simulink model "Simulacion_FIiltro_Adaptado1"  (R2020b)
settings: Solver=ode45  StartTime=0.0  StopTime=3*Tb  RelTol=1e-3  EnableMultiTasking=on
values from neighbouring files (symbols this model uses):
  Canal = 1/600    (= 0.00166666666667)    [filtroadaptado.m]
  Tb = Ts    (= 0.0276)    [filtroadaptado.m]
libraries: simulink_extras x1, commnoisgen2 x1
settings Model: Creator=Dario  LastModifiedBy=Agustin
settings DataIOCC: LimitDataPoints=on  SaveFormat=Array  ReturnWorkspaceOutputs=off
settings OptimizationCC: LifeSpan=inf
settings DebuggingCC: UnderspecifiedInitializationDetection=Classic  MergeDetectMultiDrivingBlocksExec=none  SolverPrmCheckMsg=warning  StateNameClashWarn=warning  SFUnexpectedBacktrackingDiag=warning  SFNoUnconditionalDefaultTransitionDiag=warning  SFExecutionAtInitializationDiag=none  ArithmeticOperatorsInVariantConditions=warning
settings HardwareCC: ProdBitPerPointer=32  ProdBitPerSizeT=32  ProdBitPerPtrDiffT=32  ProdLargestAtomicFloat=None  ProdIntDivRoundTo=Undefined  ProdEndianess=Unspecified  ProdWordSize=32  ProdHWDeviceType=32-bit Generic
settings ModelReferenceCC: PropagateSignalLabelsOutOfModel=off
settings SFSimCC: SimUseLocalCustomCode=off  CustomCodeUndefinedFunction=UseInterfaceOnly
settings RTWCC: RTWUseLocalCustomCode=off
settings CodeAppCC: StateflowObjectComments=on
settings GRTTargetCC: TargetLangStandard=C89/C90 (ANSI)
settings ConfigComp: CovMetricSettings=dw  CovSaveCumulativeToWorkspaceVar=on  CovSaveSingleToWorkspaceVar=on  CovExternalEMLEnable=off

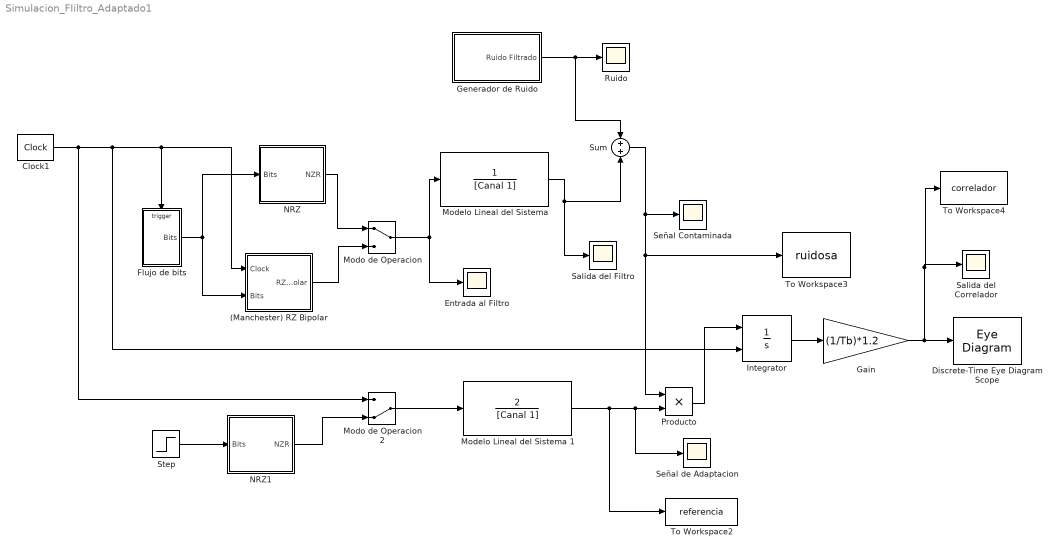
== system Simulacion_FIiltro_Adaptado1 ==
  (Manchester) RZ Bipolar : Subsystem
  Clock1 : simulink_extras/Flip Flops/Clock  period=Ts
  Discrete-Time Eye Diagram Scope : EyeDiagram  Tag=EyeDiagram
  Entrada al Filtro : Scope
  Flujo de bits : Subsystem
  Gain : Gain  Gain=(1/Tb)*1.2  SampleTime=0.001/500
  Generador de Ruido : Subsystem
  Integrator : Integrator  ExternalReset=rising
  "Modelo Lineal del Sistema " : TransferFcn  Denominator=[Canal 1]
  Modelo Lineal del Sistema 1 : TransferFcn  Numerator=[2]  Denominator=[Canal 1]
  "Modo de Operacion " : ManualSwitch
  "Modo de Operacion 2 " : ManualSwitch  CurrentSetting=0
  NRZ : Subsystem
  NRZ1 : Subsystem
  Producto : Product  RndMeth=Zero
  Ruido : Scope
  "Salida del Correlador " : Scope
  Salida del Filtro : Scope
  "Señal Contaminada " : Scope
  Señal de Adaptacion : Scope
  Step : Step  Time=0  SampleTime=0
  Sum : Sum  Inputs=+|+
  To Workspace2 : ToWorkspace  VariableName=referencia  SaveFormat=Timeseries  SampleTime=-1
  To Workspace3 : ToWorkspace  VariableName=ruidosa  SaveFormat=Timeseries  SampleTime=-1
  To Workspace4 : ToWorkspace  VariableName=correlador  SaveFormat=Timeseries  SampleTime=-1
  wires:
  Flujo de bits/1(Bits) -> (Manchester) RZ Bipolar/2(Bits), NRZ/1(Bits)
  NRZ/1(NZR) -> "Modo de Operacion "/1
  (Manchester) RZ Bipolar/1(RZ-Bipolar) -> "Modo de Operacion "/2
  "Modo de Operacion "/1 -> Entrada al Filtro/1, "Modelo Lineal del Sistema "/1
  "Modelo Lineal del Sistema "/1 -> Sum/2, Salida del Filtro/1
  Generador de Ruido/1(Ruido Filtrado) -> Ruido/1, Sum/1
  Sum/1 -> "Señal Contaminada "/1, Producto/1, To Workspace3/1
  Gain/1 -> Discrete-Time Eye Diagram Scope/1, To Workspace4/1, "Salida del Correlador "/1
  Modelo Lineal del Sistema 1/1 -> To Workspace2/1, Señal de Adaptacion/1, Producto/2
  Integrator/1 -> Gain/1
  Step/1 -> NRZ1/1(Bits)
  "Modo de Operacion 2 "/1 -> Modelo Lineal del Sistema 1/1
  Producto/1 -> Integrator/1
  Clock1/1 -> (Manchester) RZ Bipolar/1(Clock), Flujo de bits/Trigger, Integrator/2, "Modo de Operacion 2 "/1
  NRZ1/1(NZR) -> "Modo de Operacion 2 "/2

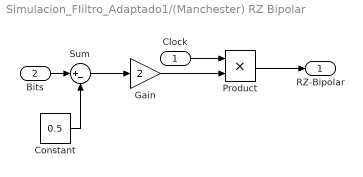
== system Simulacion_FIiltro_Adaptado1/(Manchester) RZ Bipolar ==
  Clock : Inport
  Bits : Inport  Port=2
  Constant : Constant  Value=0.5
  Gain : Gain  Gain=2
  Product : Product  RndMeth=Zero
  Sum : Sum  Inputs=|+-
  RZ-Bipolar : Outport  VectorParamsAs1DForOutWhenUnconnected=off
  wires:
  Constant/1 -> Sum/2
  Sum/1 -> Gain/1
  Gain/1 -> Product/2
  Product/1 -> RZ-Bipolar/1
  Clock/1 -> Product/1
  Bits/1 -> Sum/1

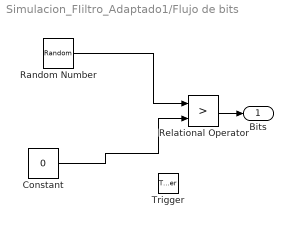
== system Simulacion_FIiltro_Adaptado1/Flujo de bits ==
  Trigger : TriggerPort  VariantControl=Variant
  Constant : Constant  Value=0
  Random Number : RandomNumber  Seed=10
  Relational Operator : RelationalOperator  Operator=>  OutDataTypeStr=boolean  RndMeth=Nearest
  Bits : Outport  VectorParamsAs1DForOutWhenUnconnected=off
  wires:
  Random Number/1 -> Relational Operator/1
  Constant/1 -> Relational Operator/2
  Relational Operator/1 -> Bits/1

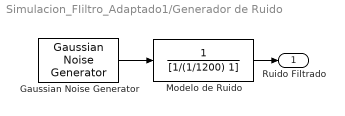
== system Simulacion_FIiltro_Adaptado1/Generador de Ruido ==
  Gaussian Noise Generator : commnoisgen2/Gaussian Noise Generator  m=0  d=varianza  s=41  Ts=0.00001  frameBased=off  sampPerFrame=1  orient=off  outDataType=double
      settings: SourceProductBaseCode=CM
  "Modelo de Ruido    " : TransferFcn  Denominator=[1/(1/1200) 1]
  Ruido Filtrado : Outport  VectorParamsAs1DForOutWhenUnconnected=off
  wires:
  Gaussian Noise Generator/1 -> "Modelo de Ruido    "/1
  "Modelo de Ruido    "/1 -> Ruido Filtrado/1

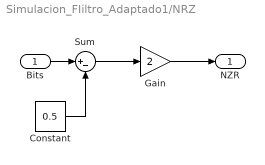
== system Simulacion_FIiltro_Adaptado1/NRZ ==
  Bits : Inport
  Constant : Constant  Value=0.5
  Gain : Gain  Gain=2
  Sum : Sum  Inputs=|+-
  NZR : Outport  VectorParamsAs1DForOutWhenUnconnected=off
  wires:
  Bits/1 -> Sum/1
  Constant/1 -> Sum/2
  Sum/1 -> Gain/1
  Gain/1 -> NZR/1

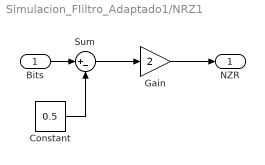
== system Simulacion_FIiltro_Adaptado1/NRZ1 ==
  Bits : Inport
  Constant : Constant  Value=0.5
  Gain : Gain  Gain=2
  Sum : Sum  Inputs=|+-
  NZR : Outport  VectorParamsAs1DForOutWhenUnconnected=off
  wires:
  Bits/1 -> Sum/1
  Constant/1 -> Sum/2
  Sum/1 -> Gain/1
  Gain/1 -> NZR/1
